simulink library "avionics_T2_lib"  (Simulink 7.2)
settings: Solver=ode45  SolverMode=SingleTasking  StartTime=0.0  StopTime=10.0  RelTol=1e-3
undefined symbols (not defined in the file or in its folder): EngineID, MAG3, Timestep
libraries: ADCgap_lib x5, simulink x4, Latency_lib x2, First_Order_Filter_lib x1, EngU2Cnt_lib x1, Cal_Loop_Table_lib x1, UDP_bus_create_lib x1, downlink_labels_lib x1, uplink_labels_lib x1
settings Model: Creator=amurch  LastModifiedBy=gtmdev

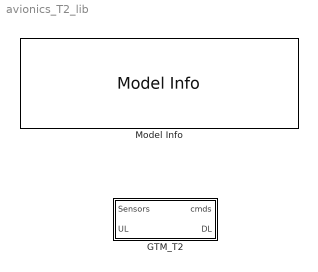
== system avionics_T2_lib ==
  GTM_T2 : Subsystem
  Model Info : simulink/Model-Wide Utilities/Model Info  SystemSampleTime=-1  InitialBlockCM=None  BlockCM=None  Frame=on  DisplayStringWithTags=|  HorizontalTextAlignment=Center  LeftAlignmentValue=0.5  SourceBlockDiagram=avionics_T2_lib  TagMaxNumber=20
      | GTM T2 Avionics Library
      | %<ModelVersion>
      | Las modified by %<LastModifiedBy> on %<LastModificationDate>

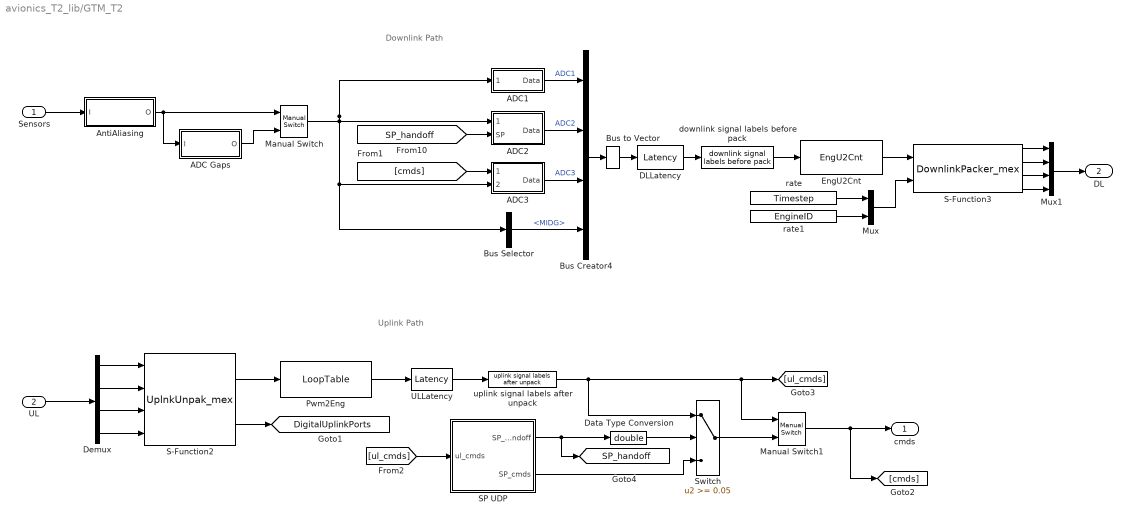
== system avionics_T2_lib/GTM_T2 ==
  note: Uplink Path
  note: Downlink Path
  Sensors : Inport  OutDataType=sfix(16)  OutScaling=2^0
  UL : Inport  Port=2  OutDataType=sfix(16)  OutScaling=2^0
  ADC Gaps : Subsystem
  ADC1 : Subsystem
  ADC2 : Subsystem
  ADC3 : Subsystem
  AntiAliasing : Subsystem
  Bus Creator4 : BusCreator
  Bus Selector : BusSelector  OutputSignals=MIDG
  Bus to Vector : BusToVector
  DLLatency : Latency_lib/Latency  SystemSampleTime=-1  Latency=.005
  Data Type Conversion : DataTypeConversion  OutDataTypeMode=double  OutDataType=sfix(16)  OutScaling=2^0  OutDataTypeStr=double  RndMeth=Nearest
  Demux : Demux
  EngU2Cnt : EngU2Cnt_lib/EngU2Cnt  SystemSampleTime=-1
  Manual Switch : simulink/Signal Routing/Manual Switch  SystemSampleTime=-1  sw=0  action=0  varsize=off
  Manual Switch1 : simulink/Signal Routing/Manual Switch  SystemSampleTime=-1  sw=0  action=0  varsize=off
  Mux : Mux  Inputs=2
  Mux1 : Mux
  Pwm2Eng : Cal_Loop_Table_lib/LoopTable  SystemSampleTime=-1  XTable=UpCals_Pwm  YTable=UpCals_Eng
  S-Function2 : S-Function  FunctionName=UplnkUnpak_mex  EnableBusSupport=off
  S-Function3 : S-Function  FunctionName=DownlinkPacker_mex  EnableBusSupport=off
  SP UDP : Subsystem
  Switch : Switch  Threshold=0.05  OutDataType=sfix(16)  OutScaling=2^0
  ULLatency : Latency_lib/Latency  SystemSampleTime=-1  Latency=.015
  downlink signal labels before pack : downlink_labels_lib/downlink signal labels before pack  SystemSampleTime=-1
  rate : Constant  Value=Timestep  OutDataType=sfix(16)  OutScaling=2^0
  rate1 : Constant  Value=EngineID  OutDataType=sfix(16)  OutScaling=2^0
  uplink signal labels after unpack : uplink_labels_lib/uplink signal labels after unpack  SystemSampleTime=-1
  cmds : Outport  OutDataType=sfix(16)  OutScaling=2^0
  DL : Outport  Port=2  OutDataType=sfix(16)  OutScaling=2^0
  tag scope: DigitalUplinkPorts=global, SP_handoff=global
  wires:
  Bus to Vector/1 -> DLLatency/1
  Sensors/1 -> AntiAliasing/1(I)
  EngU2Cnt/1 -> S-Function3/1
  rate/1 -> Mux/1
  rate1/1 -> Mux/2
  Mux/1 -> S-Function3/2
  S-Function3/1 -> Mux1/1
  S-Function3/2 -> Mux1/2
  S-Function3/3 -> Mux1/3
  S-Function3/4 -> Mux1/4
  Mux1/1 -> DL/1
  S-Function2/2 -> [DigitalUplinkPorts]
  Pwm2Eng/1 -> ULLatency/1
  Demux/1 -> S-Function2/1
  Demux/2 -> S-Function2/2
  Demux/3 -> S-Function2/3
  Demux/4 -> S-Function2/4
  UL/1 -> Demux/1
  ADC1/1(Data) -> Bus Creator4/1  "ADC1"
  ADC2/1(Data) -> Bus Creator4/2  "ADC2"
  ADC3/1(Data) -> Bus Creator4/3  "ADC3"
  Bus Selector/1 -> Bus Creator4/4  "<MIDG>"
  Bus Creator4/1 -> Bus to Vector/1
  ULLatency/1 -> uplink signal labels after unpack/1
  downlink signal labels before pack/1 -> EngU2Cnt/1
  DLLatency/1 -> downlink signal labels before pack/1
  [SP_handoff] -> ADC2/2(SP)
  [cmds] -> ADC3/1(cmds)
  S-Function2/1 -> Pwm2Eng/1
  AntiAliasing/1(O) -> Manual Switch/1, ADC Gaps/1(I)
  ADC Gaps/1(O) -> Manual Switch/2
  Manual Switch/1 -> ADC1/1(ADC1), ADC2/1(ADC2), ADC3/2(ADC3), Bus Selector/1
  uplink signal labels after unpack/1 -> Switch/1, [ul_cmds], Manual Switch1/1
  SP UDP/1(SP_handoff) -> [SP_handoff], Data Type Conversion/1
  SP UDP/2(SP_cmds) -> Switch/3
  [ul_cmds] -> SP UDP/1(ul_cmds)
  Switch/1 -> Manual Switch1/2
  Manual Switch1/1 -> cmds/1, [cmds]
  Data Type Conversion/1 -> Switch/2

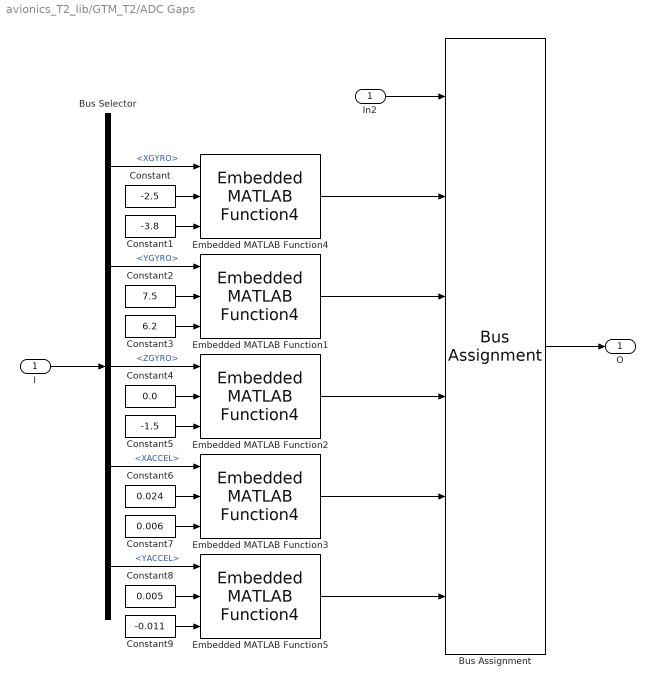
== system avionics_T2_lib/GTM_T2/ADC Gaps ==
  I : Inport  OutDataType=sfix(16)  OutScaling=2^0
  Bus Assignment : BusAssignment  AssignedSignals=MAG3.XGYRO,MAG3.YGYRO,MAG3.ZGYRO,MAG3.XACCEL,MAG3.YACCEL
  Bus Selector : BusSelector  OutputSignals=MAG3.XGYRO,MAG3.YGYRO,MAG3.ZGYRO,MAG3.XACCEL,MAG3.YACCEL
  Constant : Constant  Value=-2.5  OutDataType=sfix(16)  OutScaling=2^0
  Constant1 : Constant  Value=-3.8  OutDataType=sfix(16)  OutScaling=2^0
  Constant2 : Constant  Value=7.5  OutDataType=sfix(16)  OutScaling=2^0
  Constant3 : Constant  Value=6.2  OutDataType=sfix(16)  OutScaling=2^0
  Constant4 : Constant  Value=0.0  OutDataType=sfix(16)  OutScaling=2^0
  Constant5 : Constant  Value=-1.5  OutDataType=sfix(16)  OutScaling=2^0
  Constant6 : Constant  Value=0.024  OutDataType=sfix(16)  OutScaling=2^0
  Constant7 : Constant  Value=0.006  OutDataType=sfix(16)  OutScaling=2^0
  Constant8 : Constant  Value=0.005  OutDataType=sfix(16)  OutScaling=2^0
  Constant9 : Constant  Value=-0.011  OutDataType=sfix(16)  OutScaling=2^0
  Embedded MATLAB Function{1..5} (5 alike) : ADCgap_lib/Embedded MATLAB Function4  SystemSampleTime=-1
  In2 : InportShadow  Port=1  OutDataType=sfix(16)  OutScaling=2^0  LatchByCopyingInsideSignal=off
  O : Outport  OutDataType=sfix(16)  OutScaling=2^0
  wires:
  Bus Assignment/1 -> O/1
  Embedded MATLAB Function5/1 -> Bus Assignment/6
  Embedded MATLAB Function3/1 -> Bus Assignment/5
  Embedded MATLAB Function2/1 -> Bus Assignment/4
  Embedded MATLAB Function1/1 -> Bus Assignment/3
  Embedded MATLAB Function4/1 -> Bus Assignment/2
  In2/1 -> Bus Assignment/1
  Constant9/1 -> Embedded MATLAB Function5/3
  Constant8/1 -> Embedded MATLAB Function5/2
  Bus Selector/5 -> Embedded MATLAB Function5/1  "<YACCEL>"
  Constant7/1 -> Embedded MATLAB Function3/3
  Constant6/1 -> Embedded MATLAB Function3/2
  Bus Selector/4 -> Embedded MATLAB Function3/1  "<XACCEL>"
  Constant5/1 -> Embedded MATLAB Function2/3
  Constant4/1 -> Embedded MATLAB Function2/2
  Bus Selector/3 -> Embedded MATLAB Function2/1  "<ZGYRO>"
  Constant2/1 -> Embedded MATLAB Function1/2
  Constant3/1 -> Embedded MATLAB Function1/3
  Constant1/1 -> Embedded MATLAB Function4/3
  Constant/1 -> Embedded MATLAB Function4/2
  Bus Selector/2 -> Embedded MATLAB Function1/1  "<YGYRO>"
  Bus Selector/1 -> Embedded MATLAB Function4/1  "<XGYRO>"
  I/1 -> Bus Selector/1

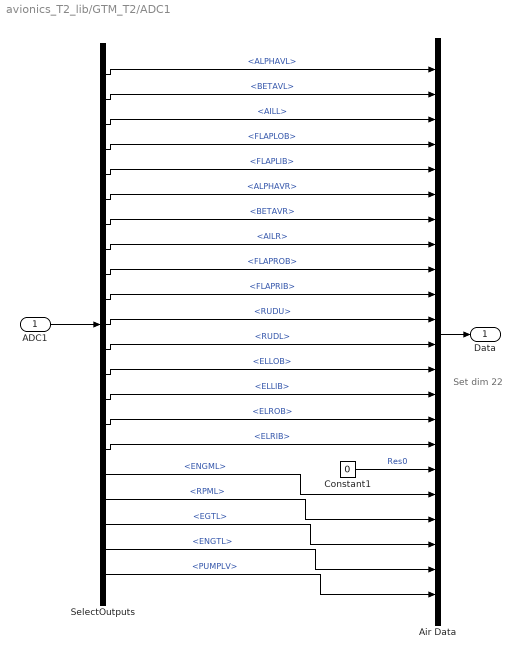
== system avionics_T2_lib/GTM_T2/ADC1 ==
  note: Set dim 22
  ADC1 : Inport  OutDataType=sfix(16)  OutScaling=2^0
  Air Data : BusCreator  Inputs=22
  Constant1 : Constant  Value=0  OutDataType=sfix(16)  OutScaling=2^0
  SelectOutputs : BusSelector  OutputSignals=Vanes.ALPHAVL,Vanes.BETAVL,Pots.AILL,Pots.FLAPLOB,Pots.FLAPLIB,Vanes.ALPHAVR,Vanes.BETAVR,Pots.AILR,Pots.FLAPROB,Pots.FLAPRIB,Pots.RUDU,Pots.RUDL,Pots.ELLOB,Pots.ELLIB,Pots.ELROB,Pots.ELRIB,ECUL.ENGML,ECUL.RPML,ECUL.EGTL,ECUL.ENGTL,ECUL.PUMPLV
  Data : Outport  PortDimensions=22  OutDataType=sfix(16)  OutScaling=2^0
  wires:
  SelectOutputs/21 -> Air Data/22  "<PUMPLV>"
  SelectOutputs/20 -> Air Data/21  "<ENGTL>"
  SelectOutputs/19 -> Air Data/20  "<EGTL>"
  SelectOutputs/18 -> Air Data/19  "<RPML>"
  SelectOutputs/17 -> Air Data/18  "<ENGML>"
  SelectOutputs/16 -> Air Data/16  "<ELRIB>"
  SelectOutputs/15 -> Air Data/15  "<ELROB>"
  SelectOutputs/14 -> Air Data/14  "<ELLIB>"
  SelectOutputs/13 -> Air Data/13  "<ELLOB>"
  SelectOutputs/12 -> Air Data/12  "<RUDL>"
  SelectOutputs/11 -> Air Data/11  "<RUDU>"
  SelectOutputs/10 -> Air Data/10  "<FLAPRIB>"
  SelectOutputs/9 -> Air Data/9  "<FLAPROB>"
  SelectOutputs/8 -> Air Data/8  "<AILR>"
  SelectOutputs/7 -> Air Data/7  "<BETAVR>"
  SelectOutputs/6 -> Air Data/6  "<ALPHAVR>"
  SelectOutputs/5 -> Air Data/5  "<FLAPLIB>"
  SelectOutputs/4 -> Air Data/4  "<FLAPLOB>"
  SelectOutputs/3 -> Air Data/3  "<AILL>"
  SelectOutputs/2 -> Air Data/2  "<BETAVL>"
  SelectOutputs/1 -> Air Data/1  "<ALPHAVL>"
  Constant1/1 -> Air Data/17  "Res0"
  Air Data/1 -> Data/1
  ADC1/1 -> SelectOutputs/1

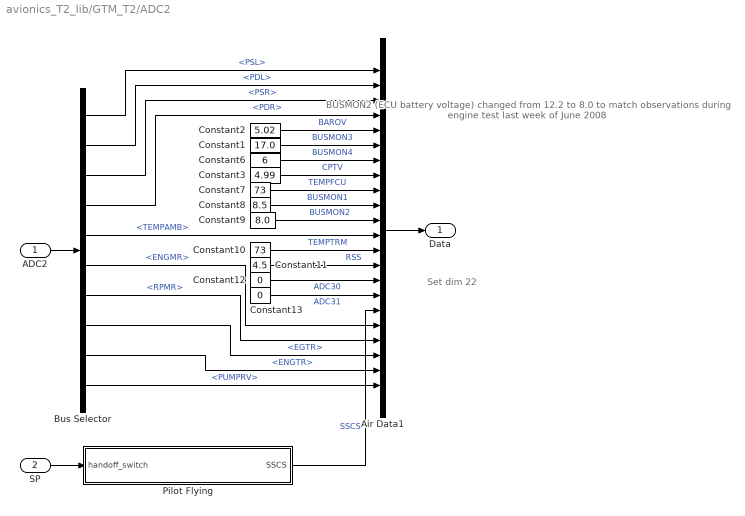
== system avionics_T2_lib/GTM_T2/ADC2 ==
  note: BUSMON2 (ECU battery voltage)
      | changed from 12.2 to 8.0 to
      | match observations during engine test
      | last week of June 2008
  note: Set dim 22
  ADC2 : Inport  OutDataType=sfix(16)  OutScaling=2^0
  SP : Inport  Port=2  OutDataType=sfix(16)  OutScaling=2^0
  Air Data1 : BusCreator  Inputs=22
  Bus Selector : BusSelector  OutputSignals=AirData.PSL,AirData.PDL,AirData.PSR,AirData.PDR,AirData.TEMPAMB,ECUR.ENGMR,ECUR.RPMR,ECUR.EGTR,ECUR.ENGTR,ECUR.PUMPRV
  Constant1 : Constant  Value=17.0  OutDataType=sfix(16)  OutScaling=2^0
  Constant10 : Constant  Value=73  OutDataType=sfix(16)  OutScaling=2^0
  Constant11 : Constant  Value=4.5  OutDataType=sfix(16)  OutScaling=2^0
  Constant12 : Constant  Value=0  OutDataType=sfix(16)  OutScaling=2^0
  Constant13 : Constant  Value=0  OutDataType=sfix(16)  OutScaling=2^0
  Constant2 : Constant  Value=5.02  OutDataType=sfix(16)  OutScaling=2^0
  Constant3 : Constant  Value=4.99  OutDataType=sfix(16)  OutScaling=2^0
  Constant6 : Constant  Value=6  OutDataType=sfix(16)  OutScaling=2^0
  Constant7 : Constant  Value=73  OutDataType=sfix(16)  OutScaling=2^0
  Constant8 : Constant  Value=8.5  OutDataType=sfix(16)  OutScaling=2^0
  Constant9 : Constant  Value=8.0  OutDataType=sfix(16)  OutScaling=2^0
  Pilot Flying : Stateflow chart
  Data : Outport  PortDimensions=22  OutDataType=sfix(16)  OutScaling=2^0
  wires:
  Air Data1/1 -> Data/1
  ADC2/1 -> Bus Selector/1
  Bus Selector/1 -> Air Data1/1  "<PSL>"
  Bus Selector/2 -> Air Data1/2  "<PDL>"
  Bus Selector/3 -> Air Data1/3  "<PSR>"
  Bus Selector/4 -> Air Data1/4  "<PDR>"
  Bus Selector/5 -> Air Data1/12  "<TEMPAMB>"
  Constant2/1 -> Air Data1/5  "BAROV"
  Constant1/1 -> Air Data1/6  "BUSMON3"
  Constant6/1 -> Air Data1/7  "BUSMON4"
  Constant3/1 -> Air Data1/8  "CPTV"
  Constant7/1 -> Air Data1/9  "TEMPFCU"
  Constant8/1 -> Air Data1/10  "BUSMON1"
  Constant9/1 -> Air Data1/11  "BUSMON2"
  Constant10/1 -> Air Data1/13  "TEMPTRM"
  Constant11/1 -> Air Data1/14  "RSS"
  Constant12/1 -> Air Data1/15  "ADC30"
  Constant13/1 -> Air Data1/16  "ADC31"
  SP/1 -> Pilot Flying/1(handoff_switch)
  Bus Selector/6 -> Air Data1/18  "<ENGMR>"
  Bus Selector/7 -> Air Data1/19  "<RPMR>"
  Bus Selector/8 -> Air Data1/20  "<EGTR>"
  Bus Selector/9 -> Air Data1/21  "<ENGTR>"
  Bus Selector/10 -> Air Data1/22  "<PUMPRV>"
  Pilot Flying/1(SSCS) -> Air Data1/17  "SSCS"

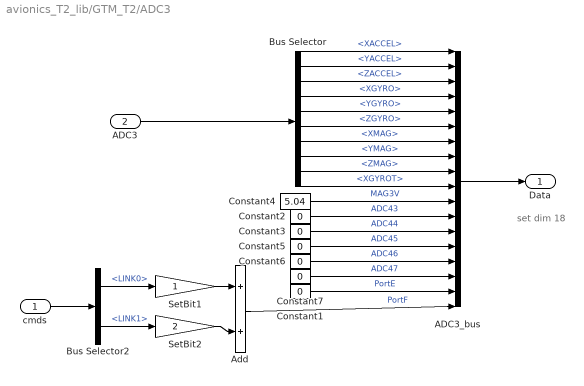
== system avionics_T2_lib/GTM_T2/ADC3 ==
  note: set dim 18
  cmds : Inport  OutDataType=sfix(16)  OutScaling=2^0
  ADC3 : Inport  Port=2  OutDataType=sfix(16)  OutScaling=2^0
  ADC3_bus : BusCreator  Inputs=18
  Add : Sum  OutDataType=sfix(16)  OutScaling=2^-10
  Bus Selector : BusSelector  OutputSignals=MAG3.XACCEL,MAG3.YACCEL,MAG3.ZACCEL,MAG3.XGYRO,MAG3.YGYRO,MAG3.ZGYRO,MAG3.XMAG,MAG3.YMAG,MAG3.ZMAG,MAG3.XGYROT
  Bus Selector2 : BusSelector  OutputSignals=LINK0,LINK1
  Constant{1..3,5..7} (6 alike) : Constant  Value=0  OutDataType=sfix(16)  OutScaling=2^0
  Constant4 : Constant  Value=5.04  OutDataType=sfix(16)  OutScaling=2^0
  SetBit1 : Gain  ParameterDataType=sfix(16)  ParameterScaling=2^0  OutDataType=sfix(16)  OutScaling=2^0  OutDataTypeStr=Inherit: Same as input
  SetBit2 : Gain  Gain=2  ParameterDataType=sfix(16)  ParameterScaling=2^0  OutDataType=sfix(16)  OutScaling=2^0  OutDataTypeStr=Inherit: Same as input
  Data : Outport  PortDimensions=18  OutDataType=sfix(16)  OutScaling=2^0
  wires:
  Constant6/1 -> ADC3_bus/15  "ADC46"
  Constant5/1 -> ADC3_bus/14  "ADC45"
  Constant3/1 -> ADC3_bus/13  "ADC44"
  Constant2/1 -> ADC3_bus/12  "ADC43"
  Add/1 -> ADC3_bus/18  "PortF"
  cmds/1 -> Bus Selector2/1
  Constant1/1 -> ADC3_bus/17  "PortE"
  ADC3_bus/1 -> Data/1
  ADC3/1 -> Bus Selector/1
  Constant4/1 -> ADC3_bus/11  "MAG3V"
  Constant7/1 -> ADC3_bus/16  "ADC47"
  Bus Selector/10 -> ADC3_bus/10  "<XGYROT>"
  Bus Selector/1 -> ADC3_bus/1  "<XACCEL>"
  Bus Selector/2 -> ADC3_bus/2  "<YACCEL>"
  Bus Selector/3 -> ADC3_bus/3  "<ZACCEL>"
  Bus Selector/4 -> ADC3_bus/4  "<XGYRO>"
  Bus Selector/5 -> ADC3_bus/5  "<YGYRO>"
  Bus Selector/6 -> ADC3_bus/6  "<ZGYRO>"
  Bus Selector/7 -> ADC3_bus/7  "<XMAG>"
  Bus Selector/8 -> ADC3_bus/8  "<YMAG>"
  Bus Selector/9 -> ADC3_bus/9  "<ZMAG>"
  Bus Selector2/1 -> SetBit1/1  "<LINK0>"
  Bus Selector2/2 -> SetBit2/1  "<LINK1>"
  SetBit1/1 -> Add/1
  SetBit2/1 -> Add/2

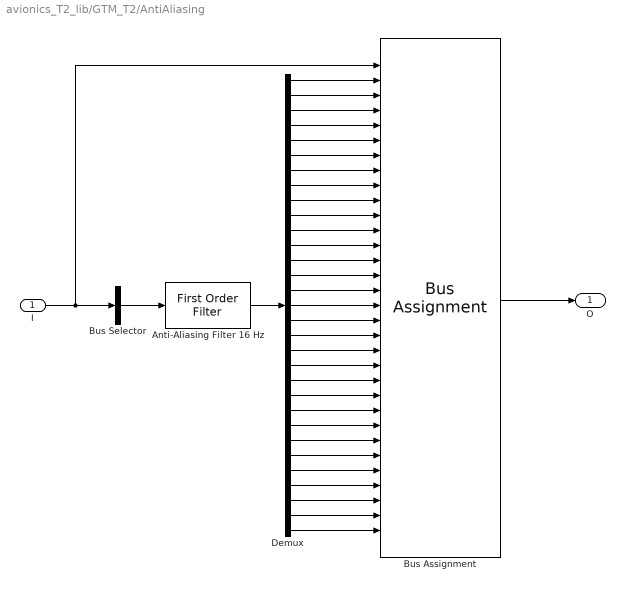
== system avionics_T2_lib/GTM_T2/AntiAliasing ==
  I : Inport  OutDataType=sfix(16)  OutScaling=2^0
  Anti-Aliasing Filter 16 Hz : First_Order_Filter_lib/First Order Filter  SystemSampleTime=-1  tau=1/(32*pi)  timestep=Timestep
  Bus Assignment : BusAssignment  AssignedSignals=Vanes.ALPHAVL,Vanes.BETAVL,Vanes.ALPHAVR,Vanes.BETAVR,AirData.PDL,AirData.PSL,AirData.PDR,AirData.PSR,AirData.TEMPAMB,MAG3.XMAG,MAG3.YMAG,MAG3.ZMAG,MAG3.XGYRO,MAG3.YGYRO,MAG3.ZGYRO,MAG3.XACCEL,MAG3.YACCEL,MAG3.ZACCEL,MAG3.XGYROT,Pots.ELLOB,Pots.ELLIB,Pots.ELROB,Pots.ELRIB,Pots.AILL,Pots.AILR,Pots.RUDU,Pots.RUDL,Pots.FLAPLIB,Pots.FLAPLOB,Pots.FLAPRIB,Pots.FLAPROB
  Bus Selector : BusSelector  OutputSignals=Vanes,AirData,MAG3,Pots  OutputAsBus=on
  Demux : Demux  Outputs=31
  O : Outport  OutDataType=sfix(16)  OutScaling=2^0
  wires:
  I/1 -> Bus Selector/1, Bus Assignment/1
  Bus Selector/1 -> Anti-Aliasing Filter 16 Hz/1
  Anti-Aliasing Filter 16 Hz/1 -> Demux/1
  Bus Assignment/1 -> O/1
  Demux/1 -> Bus Assignment/2
  Demux/2 -> Bus Assignment/3
  Demux/3 -> Bus Assignment/4
  Demux/4 -> Bus Assignment/5
  Demux/5 -> Bus Assignment/6
  Demux/6 -> Bus Assignment/7
  Demux/7 -> Bus Assignment/8
  Demux/8 -> Bus Assignment/9
  Demux/9 -> Bus Assignment/10
  Demux/10 -> Bus Assignment/11
  Demux/11 -> Bus Assignment/12
  Demux/12 -> Bus Assignment/13
  Demux/13 -> Bus Assignment/14
  Demux/14 -> Bus Assignment/15
  Demux/15 -> Bus Assignment/16
  Demux/16 -> Bus Assignment/17
  Demux/17 -> Bus Assignment/18
  Demux/18 -> Bus Assignment/19
  Demux/19 -> Bus Assignment/20
  Demux/20 -> Bus Assignment/21
  Demux/21 -> Bus Assignment/22
  Demux/22 -> Bus Assignment/23
  Demux/23 -> Bus Assignment/24
  Demux/24 -> Bus Assignment/25
  Demux/25 -> Bus Assignment/26
  Demux/26 -> Bus Assignment/27
  Demux/27 -> Bus Assignment/28
  Demux/28 -> Bus Assignment/29
  Demux/29 -> Bus Assignment/30
  Demux/30 -> Bus Assignment/31
  Demux/31 -> Bus Assignment/32

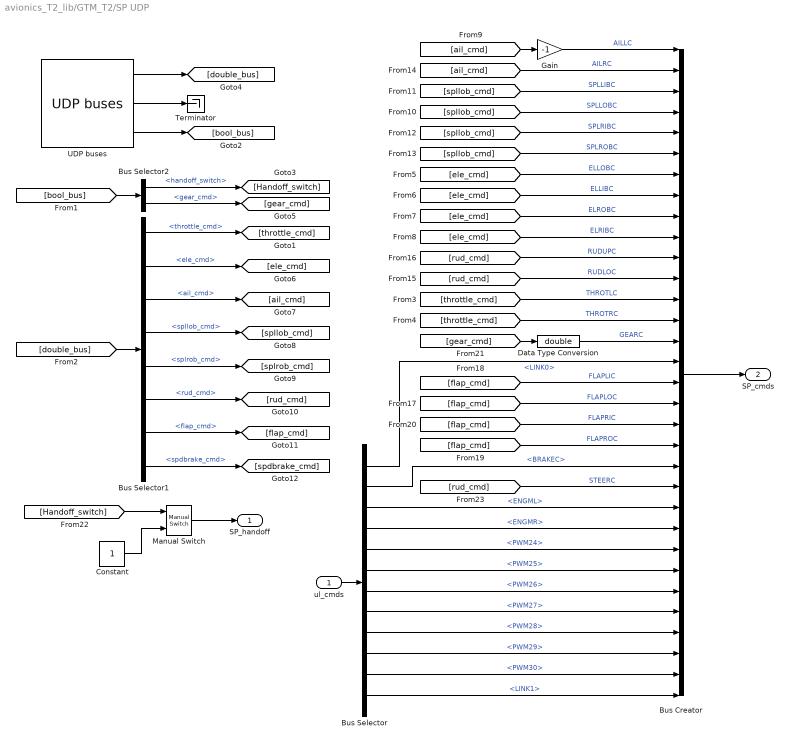
== system avionics_T2_lib/GTM_T2/SP UDP ==
  ul_cmds : Inport  OutDataType=sfix(16)  OutScaling=2^0
  Bus Creator : BusCreator  Inputs=32
  Bus Selector : BusSelector  OutputSignals=LINK0,BRAKEC,ENGML,ENGMR,PWM24,PWM25,PWM26,PWM27,PWM28,PWM29,PWM30,LINK1
  Bus Selector1 : BusSelector  OutputSignals=throttle_cmd,ele_cmd,ail_cmd,spllob_cmd,splrob_cmd,rud_cmd,flap_cmd,spdbrake_cmd
  Bus Selector2 : BusSelector  OutputSignals=handoff_switch,gear_cmd
  Constant : Constant  OutDataType=sfix(16)  OutScaling=2^0  SampleTime=-1
  Data Type Conversion : DataTypeConversion  OutDataTypeMode=double  OutDataType=sfix(16)  OutScaling=2^0  OutDataTypeStr=double
  Gain : Gain  Gain=-1  ParameterDataType=sfix(16)  ParameterScaling=2^0  OutDataType=sfix(16)  OutScaling=2^0
  Manual Switch : simulink/Signal Routing/Manual Switch  SystemSampleTime=-1  sw=1  action=0  varsize=off
  Terminator : Terminator
  UDP buses : UDP_bus_create_lib/UDP buses  SystemSampleTime=-1
  SP_handoff : Outport  OutDataType=sfix(16)  OutScaling=2^0
  SP_cmds : Outport  Port=2  OutDataType=sfix(16)  OutScaling=2^0
  wires:
  UDP buses/3 -> [bool_bus]
  UDP buses/2 -> Terminator/1
  UDP buses/1 -> [double_bus]
  [bool_bus] -> Bus Selector2/1
  Bus Selector2/1 -> [Handoff_switch]  "<handoff_switch>"
  Bus Selector2/2 -> [gear_cmd]  "<gear_cmd>"
  [double_bus] -> Bus Selector1/1
  Bus Selector1/1 -> [throttle_cmd]  "<throttle_cmd>"
  Bus Selector1/2 -> [ele_cmd]  "<ele_cmd>"
  Bus Selector1/3 -> [ail_cmd]  "<ail_cmd>"
  Bus Selector1/4 -> [spllob_cmd]  "<spllob_cmd>"
  Bus Selector1/5 -> [splrob_cmd]  "<splrob_cmd>"
  Bus Selector1/6 -> [rud_cmd]  "<rud_cmd>"
  Bus Selector1/7 -> [flap_cmd]  "<flap_cmd>"
  Bus Selector1/8 -> [spdbrake_cmd]  "<spdbrake_cmd>"
  [ail_cmd] -> Gain/1
  [gear_cmd] -> Data Type Conversion/1
  Bus Selector/3 -> Bus Creator/23  "<ENGML>"
  Bus Selector/4 -> Bus Creator/24  "<ENGMR>"
  Bus Selector/5 -> Bus Creator/25  "<PWM24>"
  Bus Selector/6 -> Bus Creator/26  "<PWM25>"
  Bus Selector/7 -> Bus Creator/27  "<PWM26>"
  Bus Selector/8 -> Bus Creator/28  "<PWM27>"
  Bus Selector/9 -> Bus Creator/29  "<PWM28>"
  Bus Selector/10 -> Bus Creator/30  "<PWM29>"
  Bus Selector/11 -> Bus Creator/31  "<PWM30>"
  Bus Selector/12 -> Bus Creator/32  "<LINK1>"
  Gain/1 -> Bus Creator/1  "AILLC"
  [ail_cmd] -> Bus Creator/2  "AILRC"
  [spllob_cmd] -> Bus Creator/3  "SPLLIBC"
  [spllob_cmd] -> Bus Creator/4  "SPLLOBC"
  [spllob_cmd] -> Bus Creator/5  "SPLRIBC"
  [spllob_cmd] -> Bus Creator/6  "SPLROBC"
  [ele_cmd] -> Bus Creator/7  "ELLOBC"
  [ele_cmd] -> Bus Creator/8  "ELLIBC"
  [ele_cmd] -> Bus Creator/9  "ELROBC"
  [ele_cmd] -> Bus Creator/10  "ELRIBC"
  [rud_cmd] -> Bus Creator/11  "RUDUPC"
  [rud_cmd] -> Bus Creator/12  "RUDLOC"
  [throttle_cmd] -> Bus Creator/13  "THROTLC"
  [throttle_cmd] -> Bus Creator/14  "THROTRC"
  Data Type Conversion/1 -> Bus Creator/15  "GEARC"
  Bus Selector/1 -> Bus Creator/16  "<LINK0>"
  [flap_cmd] -> Bus Creator/17  "FLAPLIC"
  [flap_cmd] -> Bus Creator/18  "FLAPLOC"
  [flap_cmd] -> Bus Creator/19  "FLAPRIC"
  [flap_cmd] -> Bus Creator/20  "FLAPROC"
  Bus Selector/2 -> Bus Creator/21  "<BRAKEC>"
  Bus Creator/1 -> SP_cmds/1
  ul_cmds/1 -> Bus Selector/1
  [Handoff_switch] -> Manual Switch/1
  Manual Switch/1 -> SP_handoff/1
  Constant/1 -> Manual Switch/2
  [rud_cmd] -> Bus Creator/22  "STEERC"

== matlab function GTM_T2/ADC2/Pilot Flying ==
  data: handoff_switch input double; SSCS output double
function SSCS = setSSCS(handoff_switch)
% This block supports an embeddable subset of the MATLAB language.
% See the help menu for details. 

SSCS = double(0);
RPf = uint8(0);

if (handoff_switch)
    SSCS = 6.0;  %research pilot flying (SSCS)
else
    SSCS = 4.0;  %safety pilot flying  (SSCS)
end
